simulink model "power_PSTdeltahex"  (Simulink 6.0)
settings: Solver=ode23tb  StartTime=0.0  StopTime=50  MaxStep=1/60  RelTol=1e-4  AbsTol=1e-3
undefined symbols (not defined in the file or in its folder): I21_init_imag, I21_init_real
libraries: powerlib x117, powerlib_extras x19, simulink_extras x1
(part 1 of 3)
settings Model: Creator=batserve  LastModifiedBy=batserve  ExtModeAutoUpdateStatusClock=off
settings DataIOCC: SignalLoggingName=sigsOut
settings DebuggingCC: CheckExecutionContextPreStartOutputMsg=on  CheckExecutionContextRuntimeOutputMsg=on  SolverPrmCheckMsg=none
settings HardwareCC: TargetUnknown=on

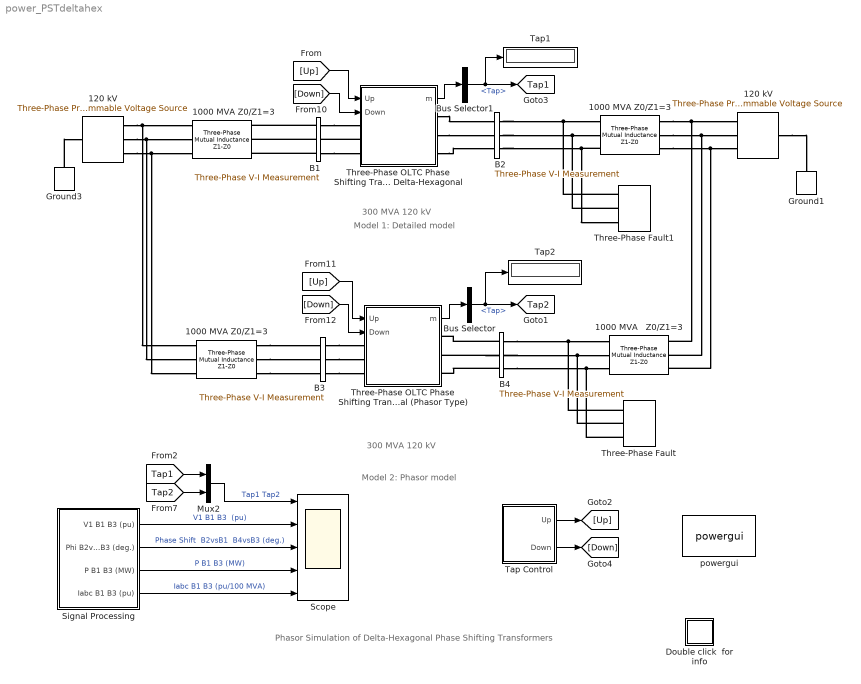
== system power_PSTdeltahex ==
  note: Phasor Simulation of Delta-Hexagonal Phase Shifting Transformers
  note: Model 1: Detailed model
  note: Model 2: Phasor model
  note: 300 MVA 120 kV
  note: 300 MVA 120 kV
  "1000 MVA Z0/Z1=3 " : powerlib/Elements/Three-Phase Mutual Inductance Z1-Z0  PhysicalDomain=powersysdomain  SubClassName=unknown  LeftPortType=p1  RightPortType=p1  LConnTagsString=a|b|c  RConnTagsString=A|B|C  PositiveSequence="[ 0.1  1/(2*pi*60)] *120e3^2/1000e6"  ZeroSequence="[ 0.3  3/(2*pi*60)] *120e3^2/1000e6"
  "1000 MVA Z0/Z1=3  " : powerlib/Elements/Three-Phase Mutual Inductance Z1-Z0  PhysicalDomain=powersysdomain  SubClassName=unknown  LeftPortType=p1  RightPortType=p1  LConnTagsString=a|b|c  RConnTagsString=A|B|C  PositiveSequence="[ 0.1  1/(2*pi*60)] *120e3^2/1000e6"  ZeroSequence="[ 0.3  3/(2*pi*60)] *120e3^2/1000e6"
  "1000 MVA Z0/Z1=3     " : powerlib/Elements/Three-Phase Mutual Inductance Z1-Z0  PhysicalDomain=powersysdomain  SubClassName=unknown  LeftPortType=p1  RightPortType=p1  LConnTagsString=a|b|c  RConnTagsString=A|B|C  PositiveSequence="[ 0.1  1/(2*pi*60)] *120e3^2/1000e6"  ZeroSequence="[ 0.3  3/(2*pi*60)] *120e3^2/1000e6"
  "1000 MVA   Z0/Z1=3       " : powerlib/Elements/Three-Phase Mutual Inductance Z1-Z0  PhysicalDomain=powersysdomain  SubClassName=unknown  LeftPortType=p1  RightPortType=p1  LConnTagsString=a|b|c  RConnTagsString=A|B|C  PositiveSequence="[ 0.1  1/(2*pi*60)] *120e3^2/1000e6"  ZeroSequence="[ 0.3  3/(2*pi*60)] *120e3^2/1000e6"
  120 kV : powerlib/Electrical Sources/Three-Phase Programmable Voltage Source  PositiveSequence=[120e3 0 60]  VariationEntity=None  VariationType=Table of time-amplitude pairs  VariationStep=0.2  VariationRate=10  VariationMagnitude=0.3  VariationFrequency=2  VariationTiming="[5  20]"  VariationPhaseA=off  Amplitudes="[ 1 0.95   1.1 ]"  TimeValues="[0  10 50]"  HarmonicGeneration=off  HarmonicA=[3 0.2 -25 0]  HarmonicB=[2 0.15 35 2]  Timing="[0.05  3]"
  "120 kV " : powerlib/Electrical Sources/Three-Phase Programmable Voltage Source  Orientation=left  PositiveSequence=[120e3 0 60]  VariationEntity=None  VariationType=Table of time-amplitude pairs  VariationStep=0.2  VariationRate=10  VariationMagnitude=0.3  VariationFrequency=2  VariationTiming="[5  20]"  VariationPhaseA=off  Amplitudes="[ 1 0.95   1.1 ]"  TimeValues="[0  10 50]"  HarmonicGeneration=off  HarmonicA=[3 0.2 -25 0]  HarmonicB=[2 0.15 35 2]  Timing="[0.05  3]"
  B1 : powerlib/Measurements/Three-Phase V-I Measurement  VoltageMeasurement=phase-to-ground  SetLabelV=on  LabelV=VabcB1  Vpu=on  Vbase=120e3  CurrentMeasurement=yes  SetLabelI=on  LabelI=IabcB1  Ipu=on  Pbase=100e6  OutputType=Complex  PhasorSimulation=on  PSBequivalent=0
  B2 : powerlib/Measurements/Three-Phase V-I Measurement  VoltageMeasurement=phase-to-ground  SetLabelV=on  LabelV=VabcB2  Vpu=on  Vbase=120e3  CurrentMeasurement=no  SetLabelI=on  LabelI=IB2  Ipu=off  Pbase=100e6  OutputType=Complex  PhasorSimulation=on  PSBequivalent=0
  B3 : powerlib/Measurements/Three-Phase V-I Measurement  VoltageMeasurement=phase-to-ground  SetLabelV=on  LabelV=VabcB3  Vpu=on  Vbase=120e3  CurrentMeasurement=yes  SetLabelI=on  LabelI=IabcB3  Ipu=on  Pbase=100e6  OutputType=Complex  PhasorSimulation=on  PSBequivalent=0
  B4 : powerlib/Measurements/Three-Phase V-I Measurement  VoltageMeasurement=phase-to-ground  SetLabelV=on  LabelV=VabcB4  Vpu=on  Vbase=120e3  CurrentMeasurement=no  SetLabelI=on  LabelI=IabcB4  Ipu=off  Pbase=100e6  OutputType=Complex  PhasorSimulation=on  PSBequivalent=0
  Bus Selector : BusSelector  DialogController=Simulink.DDGSource_Bus  OutputSignals=Tap
  Bus Selector1 : BusSelector  DialogController=Simulink.DDGSource_Bus  OutputSignals=Tap
  Double click  for info : Subsystem
      mask Display: disp('?')
  Ground1 : powerlib/Elements/Ground  Orientation=down  PhysicalDomain=powersysdomain  SubClassName=unknown  LeftPortType=p1  RightPortType=p1  LConnTagsString=a  RConnTagsString=__newr0
  Ground3 : powerlib/Elements/Ground  Orientation=down  PhysicalDomain=powersysdomain  SubClassName=unknown  LeftPortType=p1  RightPortType=p1  LConnTagsString=a  RConnTagsString=__newr0
  Mux2 : Mux  Inputs=2
  Scope : Scope  NumInputPorts=5
      settings: TimeRange=50  YMin=-5~0.94~-40~-400~0  YMax=5~1.02~40~400~3
  Signal Processing : Subsystem
      mask Display: disp('Signal\nProcessing')
  Tap Control : Subsystem
  Tap1 : Display
      settings: SampleTime=0.1
  Tap2 : Display
      settings: SampleTime=0.1
  Three-Phase Fault : powerlib/Elements/Three-Phase Fault  FaultA=off  FaultB=off  FaultC=off  FaultResistance=0.001  GroundFault=on  GroundResistance=0.001  External=off  SwitchStatus=[1 ]  SwitchTimes=[ 5 ]  InitialStates=[0 0 1]  SnubberResistance=1e6  SnubberCapacitance=inf  Measurements=None
  Three-Phase Fault1 : powerlib/Elements/Three-Phase Fault  FaultA=off  FaultB=off  FaultC=off  FaultResistance=0.001  GroundFault=on  GroundResistance=0.001  External=off  SwitchStatus=[1 ]  SwitchTimes=[ 5 ]  InitialStates=[0 0 1]  SnubberResistance=1e6  SnubberCapacitance=inf  Measurements=None
  Three-Phase OLTC Phase Shifting Transformer Delta-Hexagonal : Subsystem  mask(Phase Shifting Transformer; Delta-Hexagonal Connexion){NominalParameters=[120e3  300e6  60], RXpu=[0.15/30  0.15], RmXmpu=[500 500], SetSaturation=off, SaturationCurrentFlux=[0 0; 0.002 1.0; 0.006 1.12; 0.009 1.15; 0.015 1.17; 0.03 1.19; 0.05 1.20; 0.08 1.21; 1.0 1.302], InitialTap=0, TapSelectionTime=2.9, TransferTime=0.05, Rtransfer=1}
      mask prompts: NominalParameters "Nominal parameters [Vnom(Vrms Ph Ph) Pnom(VA)  Fnom(Hz)];"; RXpu "Resistance and leakage reactance at max. tap [R(pu)  X(pu)]"; RmXmpu "Magnetization branch [Rm(pu)  Xm(pu)]"; SetSaturation "Simulate saturation"; SaturationCurrentFlux "Saturation characteristic [i1 phi; i2 phi2; ....] (pu)"; InitialTap "Initial tap (-10 to +10)"; TapSelectionTime "Tap selection time (s) (typical 3-10 s)"; TransferTime "Tap transition time (s) (typical 40-60 ms)"; Rtransfer "Transfer resistances (ohms)"
      mask help:
      | This model implements a phase shifting transformer (PST) using the delta-hexagonal connexion. Each phase consists of two coupled windings: one fixed winding and one tapped winding (10 taps per half winding or 21 taps total). Two OLTCs are used to vary phase shift from -60 degrees to + 60 degrees by moving the transformer input connections (ABC) and output connections (abc) symmetrically  with respect to center of the tapped winding. The OLTCs move taps one step upward or downward when the signals connected to the "Up" and "Down" inputs change from 0 to 1.
      |
      | For equally spaced taps, phase shift of output voltages (abc) with respect to input voltages (ABC) varies as follows:
      |     Psi= 2*atan(-tap/10/sqrt(3))
      | where:
      |    tap= position of the 2 OLTCs (-10<= tap<= 10)
      |
      | Tap = [0    1      2        3        4         5       6      7       8       9        10  ]
      | Phi  = [0   -6.6  -13.2  -19.7  -26.0  -32.2 -38.2 -44.0 -49.6.-54.9  -60.0]
      mask init:
      | NumberOfTaps=10;
      | if abs(InitialTap)>NumberOfTaps,
      |    h=errordlg(sprintf('The initial tap number must be an integer comprised between % d and %d',-NumberOfTaps,NumberOfTaps),'Parameter error');
      |    uiwait(h);
      | end
      | 
      | % Saturation
      | set_param([gcb,'/TransfoA'],'SetSaturation',SetSaturation);
      | set_param([gcb,'/TransfoB'],'SetSaturation',SetSaturation);
      | set_param([gcb,'/TransfoC'],'SetSaturation',SetSaturation);
      mask CallbackString:
      | |||tempMaskVis=get_param(gcb,'MaskVisibilities');
      | if strcmp(get_param(gcb,'SetSaturation'),'on')
      | 	tempMaskVis{5}='on';
      | 	set_param(gcb,'MaskVisibilities',tempMaskVis);
      | else
      | 	tempMaskVis{5}='off';
      | 	set_param(gcb,'MaskVisibilities',tempMaskVis);
      | end|||||
  Three-Phase OLTC Phase Shifting Transformer Delta-Hexagonal (Phasor Type) : Subsystem  mask(Phase Shifting Transformer; Delta-Hexagonal Connexion (phasor)){NominalParameters=[120e3  300e6  60], RXpu=[0.15/30  0.15], RXm=[500 500], NumberOfTaps=10, InitialTap=0, TapSelectionTime=2.9, Iout_init=[ 0  0]}
      mask prompts: NominalParameters "Nominal parameters [Vnom(Vrms Ph Ph) Pnom(VA)  Fnom(Hz)];"; RXpu "Resistance and leakage reactance at max. tap [R(pu)  X(pu)]"; RXm "Magnetization branch [Rm(pu)  Xm(pu)]"; NumberOfTaps "Number of taps per half tapped winding"; InitialTap "Initial tap"; TapSelectionTime "Tap selection time (s) (typical 3-10 s)"; Iout_init "Initial pos. seq. of output currents [Mag(pu)  Phase(deg)]"
      mask help:
      | This model implements a phasor model of a phase shifting transformer (PST) using the delta-hexagonal connexion. Each phase consists of two coupled windings: one fixed winding and one tapped winding. Two OLTCs are used to vary phase shift from -60 degrees to + 60 degrees
      | by moving the transformer input connections (ABC) and output connections (abc) symmetrically with respect to center of the tapped winding. The OLTCs move taps one step upward or downward when the signals connected to the "Up" and "Down" inputs change from 0 to 1.
      |
      | Phase shift Psi of output voltages (abc) with respect to input voltages (ABC) varies as follows:
      |     Psi= 2*atan(-k/sqrt(3))
      | where:
      |    k= tap position of the 2 OLTCs with respect to center of tapped winding
      |         k= tap/NumberOfTaps  ( -1<= k<= 1)
      |    k=0 indicates taps at winding mid point (Psi=0)
      |    k= 1 --> Psi=-60 deg;  k=-1--> Psi = -60 deg.
      mask init:
      | if abs(InitialTap)>NumberOfTaps
      |    h=errordlg(sprintf('The initial tap number must be an integer comprised between % d and %d',-NumberOfTaps,NumberOfTaps),'Parameter error');
      |    uiwait(h);
      | end
      | Vnom=NominalParameters(1);
      | Pnom=NominalParameters(2);
      | Fnom=NominalParameters(3);
      | w=2*pi*Fnom;
      | Ibase=Pnom/Vnom/sqrt(3)*sqrt(2);
      | 
      | TapMinMax=[-NumberOfTaps NumberOfTaps];
      | 
      | j=sqrt(-1);
      | a=exp(j*2*pi/3);
      | Z1pu=RXpu(1)+j*RXpu(2);     % Impedance at max tap position
      | Zmpu=(RXm(1)*j*RXm(2))/(RXm(1)+j*RXm(2)); % Magnetization Impedance at max tap position
      | 
      | I2_init_mag=Iout_init(1); % Mag pos. seq. (pu)
      | I2_init_pha=Iout_init(2); % Phase pos. seq. (deg)
      | I2A_init_mag=I2_init_mag*Ibase;
      | I2B_init_mag=I2_init_mag*Ibase;
      | I2C_init_mag=I2_init_mag*Ibase;
      | I2A_init_pha=I2_init_pha;
      | I2B_init_pha=I2_init_pha-120;
      | I2C_init_pha=I2_init_pha+120;
      | 
      | psi=2*atan(-InitialTap/NumberOfTaps/sqrt(3))*180/pi; % degrees
      | 
      | I1A_init_mag=I2A_init_mag;
      | I1B_init_mag=I2B_init_mag;
      | I1C_init_mag=I2C_init_mag;
      | I1A_init_pha=I2A_init_pha-psi;
      | I1B_init_pha=I2B_init_pha-psi;
      | I1C_init_pha=I2C_init_pha-psi;
      | 
      | %Initialisation of pos. seq. transfer functions for breaking alg. loop
      | [I21_init_real, I21_init_imag]=pol2cart(I2_init_pha*pi/180,I2_init_mag);
  powergui : powerlib/powergui  Priority=2  Frange=[0:2:500]  Ylog=off  Xlog=on  save=off  variable=ZData  ZoomFFT=on  StartTime=0.0  cycles=1  DisplayStyle=1  fundamental=60  FreqAxis=off  MaxFrequency=1000  frequencyindice=1  frequencyindicesteady=1  RmsSteady=2  display=off  Ts=0  methode=on  frequency=60  echomessages=off
  tag scope: Tap1=global, Tap2=global
  wires:
  [Tap1] -> Mux2/1
  [Tap2] -> Mux2/2
  Mux2/1 -> Scope/1  "Tap1 Tap2"
  Tap Control/1(Up) -> [Up]
  Tap Control/2(Down) -> [Down]
  Signal Processing/4(Iabc B1 B3 (pu)) -> Scope/5  "Iabc B1 B3 (pu/100 MVA)"
  Signal Processing/1(V1 B1 B3 (pu)) -> Scope/2  "V1 B1 B3  (pu)"
  Signal Processing/2(Phi B2vsB1  B4vsB3 (deg.)) -> Scope/3  "Phase Shift  B2vsB1  B4vsB3 (deg.)"
  Signal Processing/3(P B1 B3 (MW)) -> Scope/4  "P B1 B3 (MW)"
  Three-Phase OLTC Phase Shifting Transformer Delta-Hexagonal (Phasor Type)/1(m) -> Bus Selector/1
  Bus Selector/1 -> [Tap2], Tap2/1  "<Tap>"
  Three-Phase OLTC Phase Shifting Transformer Delta-Hexagonal/1(m) -> Bus Selector1/1
  Bus Selector1/1 -> [Tap1], Tap1/1  "<Tap>"
  [Down] -> Three-Phase OLTC Phase Shifting Transformer Delta-Hexagonal/2(Down)
  [Down] -> Three-Phase OLTC Phase Shifting Transformer Delta-Hexagonal (Phasor Type)/2(Down)
  [Up] -> Three-Phase OLTC Phase Shifting Transformer Delta-Hexagonal (Phasor Type)/1(Up)
  [Up] -> Three-Phase OLTC Phase Shifting Transformer Delta-Hexagonal/1(Up)
  connections:
  Three-Phase OLTC Phase Shifting Transformer Delta-Hexagonal/LConn2 -- B1/RConn2
  Ground3/LConn1 -- 120 kV/LConn1
  B1/RConn1 -- Three-Phase OLTC Phase Shifting Transformer Delta-Hexagonal/LConn1
  B1/RConn3 -- Three-Phase OLTC Phase Shifting Transformer Delta-Hexagonal/LConn3
  B3/RConn1 -- Three-Phase OLTC Phase Shifting Transformer Delta-Hexagonal (Phasor Type)/LConn1
  B3/RConn2 -- Three-Phase OLTC Phase Shifting Transformer Delta-Hexagonal (Phasor Type)/LConn2
  B3/RConn3 -- Three-Phase OLTC Phase Shifting Transformer Delta-Hexagonal (Phasor Type)/LConn3
  B1/LConn1 -- "1000 MVA Z0/Z1=3 "/RConn1
  B1/LConn2 -- "1000 MVA Z0/Z1=3 "/RConn2
  B1/LConn3 -- "1000 MVA Z0/Z1=3 "/RConn3
  "1000 MVA Z0/Z1=3  "/RConn1 -- B3/LConn1
  "1000 MVA Z0/Z1=3  "/RConn2 -- B3/LConn2
  "1000 MVA Z0/Z1=3  "/RConn3 -- B3/LConn3
  "1000 MVA   Z0/Z1=3       "/RConn1 -- "120 kV "/RConn1 -- "1000 MVA Z0/Z1=3     "/RConn1
  "120 kV "/LConn1 -- Ground1/LConn1
  "1000 MVA   Z0/Z1=3       "/RConn2 -- "120 kV "/RConn2 -- "1000 MVA Z0/Z1=3     "/RConn2
  "1000 MVA   Z0/Z1=3       "/RConn3 -- "120 kV "/RConn3 -- "1000 MVA Z0/Z1=3     "/RConn3
  Three-Phase OLTC Phase Shifting Transformer Delta-Hexagonal/RConn2 -- B2/LConn2
  Three-Phase OLTC Phase Shifting Transformer Delta-Hexagonal/RConn1 -- B2/LConn1
  Three-Phase OLTC Phase Shifting Transformer Delta-Hexagonal/RConn3 -- B2/LConn3
  B4/LConn1 -- Three-Phase OLTC Phase Shifting Transformer Delta-Hexagonal (Phasor Type)/RConn1
  B4/LConn2 -- Three-Phase OLTC Phase Shifting Transformer Delta-Hexagonal (Phasor Type)/RConn2
  B4/LConn3 -- Three-Phase OLTC Phase Shifting Transformer Delta-Hexagonal (Phasor Type)/RConn3
  120 kV/RConn1 -- "1000 MVA Z0/Z1=3 "/LConn1 -- "1000 MVA Z0/Z1=3  "/LConn1
  120 kV/RConn2 -- "1000 MVA Z0/Z1=3 "/LConn2 -- "1000 MVA Z0/Z1=3  "/LConn2
  120 kV/RConn3 -- "1000 MVA Z0/Z1=3 "/LConn3 -- "1000 MVA Z0/Z1=3  "/LConn3
  Three-Phase Fault/LConn3 -- "1000 MVA   Z0/Z1=3       "/LConn3 -- B4/RConn3
  Three-Phase Fault/LConn2 -- "1000 MVA   Z0/Z1=3       "/LConn2 -- B4/RConn2
  Three-Phase Fault/LConn1 -- "1000 MVA   Z0/Z1=3       "/LConn1 -- B4/RConn1
  B2/RConn3 -- "1000 MVA Z0/Z1=3     "/LConn3 -- Three-Phase Fault1/LConn3
  B2/RConn1 -- Three-Phase Fault1/LConn1 -- "1000 MVA Z0/Z1=3     "/LConn1
  B2/RConn2 -- Three-Phase Fault1/LConn2 -- "1000 MVA Z0/Z1=3     "/LConn2

== system power_PSTdeltahex/Double click  for info ==
  note: This demonstration illustrates operation of two models of Phase Shifting Transformer (PST) using On Load Tap Changers (OLTC)
  note: Circuit Description
  note: Two 120 kV 1000 MVA networks are interconnected through a phase shifting transformer (PST) . The phase shift can be varied on load  by means of On Load Tap Changers (OLTC).
      | The same circuit is duplicated in order to compare the performance of  two different models of PST:
      |
      |     - Model 1 is a detailed model where all OLTC switches and transformer characteristics are represented. This model can be used with either continuous or discrete
      |        solvers to get detailed waveshapes or with the phasor simulation method to observe variations of  phasor voltages and currents.
      |     - Model 2 is a simplified phasor model where the transformer and the OLTCs are simulated by current sources. This model can be used only with the phasor solution method
      |        The phasor model is much faster to execute and it should be the preferred model for transient stability studies.
      |
      | Both models implement a three-phase phase PST rated 120 kV, 300 MVA, and using the delta-hexagonal connection.
      | The PSTs are used to control the power transferred between the two 120 kV networks.
      |
      | Each phase consists of two coupled windings (one winding without taps, and one tapped winding). Two OLTCs are used to vary phase shift  from -60 degrees to + 60 degrees
      | by moving the transformer input connections (ABC) and  output connections (abc) symmetrically  with respect to center of the tapped winding. Each OLTC consists of ten (10)
      | switches allowing selection of  tap position -10 to +10. Taps +10 and -10 provide respectively -60 degrees and + 60 degrees phase shift of abc voltages with respect to ABC,
      | while tap 0 provides zero phase shift. With 10 taps per half winding, each tap provides approximately 6 degrees phase shift. The phase shift variation as function of tap position
      | is given in the block menu. When pulses are sent at the "Up" or  "Down" inputs, the taps move either in the positive or negative direction.
      |
      | Open the two PST block menus and look at  their parameters. The detailed model is buit with a fixed number of taps (10) whereas the phasor model allows specifying any number
      | of taps. Simulation of saturation is permitted with the detailed model only, providing that a phasor solution method is not used (specify "Continuous" or "Discretize electrical model"
      | in the powergui block).
      |
      | You can also use 'Edit/Look under mask' to see how the transformer models are built. The detailed model is built from three Multi-Winding Transformer blocks and
      | three OLTC subsystems which contain switches performing  tap selection and reversal of the regulation winding. The tap transition is performed by temporarily
      | short-circuiting two adjacent transformer taps through resistors (1 ohm resistances and 50 ms transition time as specified in the block menu of the detailed model).
      | The phasor model is built with current sources emulating the transformer impedance which depends on winding resistances, leakage reactances and tap position.
  note: G. Sybille (Hydro-Quebec)
  note: In order to observe impact of phase shift on power transfer, the phase shift is increased from zero to 32.2 degrees lagging (tap +5), then phase shift is reduced
      | to zero and increased again up to 32.2 degrees leading. This is performed by sending 5 pulses to the "Up" input, and then, 10 pulses to the "Down" input ".
      | As the tap selection is a relatively slow mechanical process (3 sec per tap as specified in the "Tap selection time" parameter of the block menus), the simulation Stop time
      | is set to 50 s.
      |
      | Start simulation and observe PST operation on the Scope. Results obtained with the two models are superimposed on five traces.
      | Trace 1 shows the tap position. Trace 2 shows a superposition of positive-sequence voltages measured at bus B1 (yellow) and bus B3 (magenta) .
      | Traces 3 shows the phase shifts of positive-sequence voltages measured at output terminals (abc) with respect to input terminals (ABC).
      | Trace 4 compares the active power measured at bus B1(yellow) and bus B3 (magenta). Trace 5 ...
      |
      | When simulation starts the OLTCs are at position 0 (zero phase shift).  As the two networks are symmetrical with both internal angles set at 0 degree,  there is no current flowing.
      | Then, phase shift is increased and bus B2 (or  B4) is lagging bus B1(or B3).  As B2 is lagging the internal voltage of the source located on right side, power flows from
      | right to left. Power measured from left to right is therefore negative for positive tap positions.
      | The maximum power is obtained at tap +5, or -5 when the phase shift is respectively -32.2 degrees and +32.2 degrees.
      | The active power can be computed from P= V1.V2*sin(psi)/ (X1 +X2 + Xpst) , where: V1=V2=internal voltages= 1.0 pu ;  X1= X2 = network reactances =  1pu /1000 MVA
      | Xpst= PST leakage reactance at tap 5. The PST leakage reactance varies vith tap position (from zero at tap zero to 0.15 pu at maximum tap (10)).
      | The positive-sequence impedance of the phasor model is available as a signal at its measurement output "m". The reactance obtained at tap 5 is  Xpst=0.1067 pu/ 300 MVA.
      | The total reactance expressed in pu/100 MVA is X= 0.1 +0.1 + 0.1067/3 =0.2356 pu/100 MVA.
      | The expected active power at tap 5 is P= 1*sin(32.2deg)/0.2356 = 2.26 pu/100 MVA or 226 MW, which corresponds well with the measured value on trace 4 (224 MW)
      | Because of the voltage developed across the PST leakage reactance, the phase shift measured between PST input and output voltages (trace 3) is lower than the expected value.
      | For example, 27.2 degrees is obtained at tap 5, instead of the 32.2 degrees theoretical value computed at no load. The phase shift variation depends on load current.
  note: Demonstration
  note: Simulation with phasor model only
  note: In order to appreciate the gain in simulation speed provided by the phasor model, delete the detailed PST model and replace it with a duplicate of the phasor model.
      | Reconnect control signals to the "Up" and  "Down" inputs. Restart simulation. The model runs approximately 5 times faster, mainly because the OLTC switches of the
      | detailed model are not simulated.
  note: Open loop control of power transfer
  note: Initializating the phasor model
  note: For the phasor model to start initialized at t=0, the current sources used in the model must be inialized with current values corresponding to steady state.
      | Suppose that you want to start with the initial tap position 5. First, in the two block menus, "set Initial tap" parameter to 5. Then disconnect the signals connected to the
      | "Up" and   "Down" inputs of the two models, so that the taps stay at position 5.  If you start simulation you will notice a transient in the phasor model signals at  t=0 because
      | the model is not initialized. Use the "Steady-State Voltages and Currents" option of the powergui to obtain the initial current flowing in the detailed model at bus B4.
      | The phase  A output current identified "B2/Ia" is 1129.4 A rms, 169 degrees. This current converted to per unit based on PST rating is 1129/1443 = 0.7824 pu/ 300MVA.
      | Specify [ 0.7824 169]  in the "Initial pos. seq. output current" parameter. If you now restart simulation, you should observe no transient at t=0.
  note: Operation under unbalanced conditions
  note: The phasor model is valid for unbalanced conditions. If you check "Phase A Fault" in the the two fault breakers, a single-phase fault will be applied at t=5s.
      | The currents measured at buses B1and B3 should be identical. (Ia=3.48 pu, Ib=2.25 pu  Ic=2.10 pu at tap position +5).

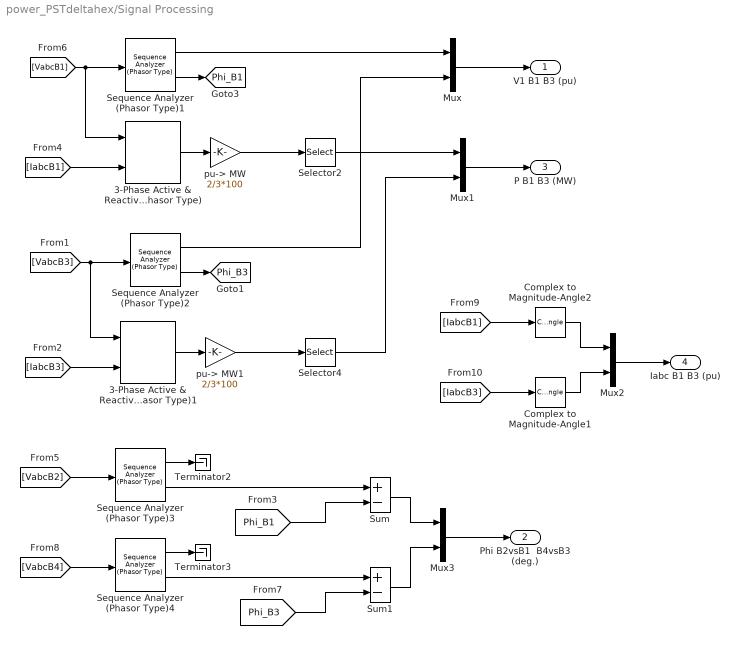
== system power_PSTdeltahex/Signal Processing ==
  3-Phase Active & Reactive Power (Phasor Type) : powerlib_extras/Phasor Library/3-Phase Active & Reactive Power (Phasor Type)
  3-Phase Active & Reactive Power (Phasor Type)1 : powerlib_extras/Phasor Library/3-Phase Active & Reactive Power (Phasor Type)
  Complex to Magnitude-Angle1 : ComplexToMagnitudeAngle  Output=Magnitude
  Complex to Magnitude-Angle2 : ComplexToMagnitudeAngle  Output=Magnitude
  Mux{,1..3} (4 alike) : Mux  Inputs=2
  Selector2 : Selector  InputPortWidth=2
  Selector4 : Selector  InputPortWidth=2
  Sequence Analyzer (Phasor Type){1..4} (4 alike) : powerlib_extras/Phasor Library/Sequence Analyzer (Phasor Type)  seq=Positive
  Sum : Sum  Inputs=+-  SaturateOnIntegerOverflow=on
  Sum1 : Sum  Inputs=+-  SaturateOnIntegerOverflow=on
  Terminator2 : Terminator
  Terminator3 : Terminator
  pu-> MW : Gain  Gain=2/3*100  SaturateOnIntegerOverflow=on
  pu-> MW1 : Gain  Gain=2/3*100  SaturateOnIntegerOverflow=on
  V1 B1 B3 (pu) : Outport
  Phi B2vsB1  B4vsB3 (deg.) : Outport  Port=2
  P B1 B3 (MW) : Outport  Port=3
  Iabc B1 B3 (pu) : Outport  Port=4
  tag scope: Phi_B1=global, Phi_B3=global
  wires:
  [VabcB1] -> Sequence Analyzer (Phasor Type)1/1, 3-Phase Active & Reactive Power (Phasor Type)/1
  Sequence Analyzer (Phasor Type)1/2 -> [Phi_B1]
  3-Phase Active & Reactive Power (Phasor Type)/1 -> pu-> MW/1
  3-Phase Active & Reactive Power (Phasor Type)1/1 -> pu-> MW1/1
  pu-> MW/1 -> Selector2/1
  pu-> MW1/1 -> Selector4/1
  [VabcB3] -> Sequence Analyzer (Phasor Type)2/1, 3-Phase Active & Reactive Power (Phasor Type)1/1
  Sequence Analyzer (Phasor Type)2/1 -> Mux/2
  Sequence Analyzer (Phasor Type)2/2 -> [Phi_B3]
  [IabcB1] -> 3-Phase Active & Reactive Power (Phasor Type)/2
  [IabcB3] -> 3-Phase Active & Reactive Power (Phasor Type)1/2
  Sequence Analyzer (Phasor Type)1/1 -> Mux/1
  Mux/1 -> V1 B1 B3 (pu)/1
  Mux1/1 -> P B1 B3 (MW)/1
  Selector2/1 -> Mux1/1
  Selector4/1 -> Mux1/2
  Sequence Analyzer (Phasor Type)3/2 -> Sum/1
  [Phi_B1] -> Sum/2
  Sequence Analyzer (Phasor Type)3/1 -> Terminator2/1
  [VabcB2] -> Sequence Analyzer (Phasor Type)3/1
  Sequence Analyzer (Phasor Type)4/2 -> Sum1/1
  [Phi_B3] -> Sum1/2
  Sequence Analyzer (Phasor Type)4/1 -> Terminator3/1
  [VabcB4] -> Sequence Analyzer (Phasor Type)4/1
  Sum/1 -> Mux3/1
  Sum1/1 -> Mux3/2
  Mux3/1 -> Phi B2vsB1  B4vsB3 (deg.)/1
  [IabcB1] -> Complex to Magnitude-Angle2/1
  Complex to Magnitude-Angle2/1 -> Mux2/1
  Mux2/1 -> Iabc B1 B3 (pu)/1
  [IabcB3] -> Complex to Magnitude-Angle1/1
  Complex to Magnitude-Angle1/1 -> Mux2/2

== system power_PSTdeltahex/Tap Control ==
  Product : Product  SaturateOnIntegerOverflow=on
  Product1 : Product  SaturateOnIntegerOverflow=on
  Pulse Generator : DiscretePulseGenerator  PulseType=Time based  Period=3  PulseWidth=5
  Pulse Generator1 : DiscretePulseGenerator  PulseType=Time based  Period=3  PulseWidth=5
  Timer1 : powerlib_extras/Control  Blocks/Timer  t="[ 0  16   ]"  e="[1   0   ]"
  Timer2 : powerlib_extras/Control  Blocks/Timer  t="[ 0  17  47 ]"  e="[0  1   0  ]"
  Up : Outport
  Down : Outport  Port=2
  wires:
  Pulse Generator/1 -> Product/1
  Timer1/1 -> Product/2
  Pulse Generator1/1 -> Product1/1
  Timer2/1 -> Product1/2
  Product1/1 -> Down/1
  Product/1 -> Up/1

== system power_PSTdeltahex/Three-Phase OLTC Phase Shifting Transformer Delta-Hexagonal ==
  Up : Inport  Port=1  LatchInput=off
  Down : Inport  Port=2  LatchInput=off
  Goto Tag Visibility : GotoTagVisibility  GotoTag=SwSelect
  Goto Tag Visibility1 : GotoTagVisibility  GotoTag=SwTransfer
  Goto Tag Visibility2 : GotoTagVisibility  GotoTag=SwInversion
  Mux : Mux  Inputs=2
  OLTC Control : Subsystem  mask{NumberOfTaps=NumberOfTaps, TapSelectorTime=TapSelectionTime, TransferSwitchTime=TransferTime, InitialTap=InitialTap}
      mask prompts: NumberOfTaps "Number of taps:"; TapSelectorTime "Operating time of the tap selector (typical 3-10 s):"; TransferSwitchTime "Operating time of the transfer switch (typical 40-60 ms):"; InitialTap "Initial tap:"
      mask init:
      | TapVector=0:2*NumberOfTaps;
      | InitialStates1=zeros(1,2*NumberOfTaps+1);
      | InitialStates1(NumberOfTaps+abs(InitialTap)+1)=1;
      | InitialStates2=zeros(1,2*NumberOfTaps+1);
      | InitialStates2(NumberOfTaps-abs(InitialTap)+1)=1;
  Subsystem1 : Subsystem
      mask Display: disp('Double click\nto see\nTransforner\nConnections')
  TransfoA : Subsystem  mask{NominalParameters=NominalParameters, RXpu=RXpu, RmXmpu=RmXmpu, SetSaturation=off, SaturationCurrentFlux=SaturationCurrentFlux, NumberOfTaps=NumberOfTaps, InitialTap=InitialTap, R=Rtransfer}
      mask prompts: NominalParameters "Nominal parameters [Vnom(Vrms Ph Ph) Pnom(VA)  Fnom(Hz)];"; RXpu "Resistance and leakage reactance at max. tap [R(pu)  X(pu)]"; RmXmpu "Magnetization branch [Rm(pu)  Xm(pu)]"; SetSaturation "Simulate saturation"; SaturationCurrentFlux "Saturation characteristic [i1 phi; i2 phi2; ....] (pu)"; NumberOfTaps "Number of taps"; InitialTap "Initial tap (-10 to +10)"; R "Transfer resistances (ohms)"
      mask init:
      | VnomLL=NominalParameters(1); % Tension LL nominale
      | Pnom3ph=NominalParameters(2);
      | Fnom=NominalParameters(3);
      | N=NumberOfTaps*2;
      | Ron=1e-4; % Resistance des interrupteurs
      | Rsnub=1e6;% Resistance des snubbers aux bornes des interrupteurs
      | 
      | % Tension nominale de chaque enroulement
      | % = Tension max. par enroulement obtenu a la prise 0
      | % =VLN_nom*2/sqrt(3)  --> Vnominal enroulements=Vnom*2/3 
      | Vnom_Windings=[VnomLL*2/3, VnomLL*2/3];
      | % RXpu= R et X des 2 enroulements en pu sur Pnom3ph et VnomLL
      | % RXpunom= R et X de chaque enroulement 
      | % en pu sur tension nominale des enroulements (VnomLL*2/3)  et Pnom3ph/3
      | RXpunom=RXpu/2*9/4; 
      | Rpu_Windings=[RXpunom(1), RXpunom(1)];
      | Xpu_Windings=[RXpunom(2), RXpunom(2)];
      | 
      | % RmXmpu= Rm et Xm en pu sur tension nominale des enroulements (VnomLL*2/3)et Pnom3ph/3  
      | Rmag=RmXmpu(1);
      | Lmag=RmXmpu(2);
      | 
      | % Saturation
      | set_param([gcb,'/Transformer'],'SetSaturation',SetSaturation)
      | 
      | InitialStates1=zeros(1,N+1);
      | InitialStates1(NumberOfTaps+abs(InitialTap)+1)=1;
      | InitialStates2=zeros(1,N+1);
      | InitialStates2(NumberOfTaps-abs(InitialTap)+1)=1;
      | InitialStates=InitialStates1|InitialStates2;
  TransfoB : Subsystem  mask{NominalParameters=NominalParameters, RXpu=RXpu, RmXmpu=RmXmpu, SetSaturation=off, SaturationCurrentFlux=SaturationCurrentFlux, NumberOfTaps=NumberOfTaps, InitialTap=InitialTap, R=Rtransfer}
      mask prompts: NominalParameters "Nominal parameters [Vnom(Vrms Ph Ph) Pnom(VA)  Fnom(Hz)];"; RXpu "Resistance and leakage reactance at max. tap [R(pu)  X(pu)]"; RmXmpu "Magnetization branch [Rm(pu)  Xm(pu)]"; SetSaturation "Simulate saturation"; SaturationCurrentFlux "Saturation characteristic [i1 phi; i2 phi2; ....] (pu)"; NumberOfTaps "Number of taps"; InitialTap "Initial tap (-10 to +10)"; R "Transfer resistances (ohms)"
      mask init: same as power_PSTdeltahex/Three-Phase OLTC Phase Shifting Transformer Delta-Hexagonal/TransfoA
  TransfoC : Subsystem  mask{NominalParameters=NominalParameters, RXpu=RXpu, RmXmpu=RmXmpu, SetSaturation=off, SaturationCurrentFlux=SaturationCurrentFlux, NumberOfTaps=NumberOfTaps, InitialTap=InitialTap, R=Rtransfer}
      mask prompts: NominalParameters "Nominal parameters [Vnom(Vrms Ph Ph) Pnom(VA)  Fnom(Hz)];"; RXpu "Resistance and leakage reactance at max. tap [R(pu)  X(pu)]"; RmXmpu "Magnetization branch [Rm(pu)  Xm(pu)]"; SetSaturation "Simulate saturation"; SaturationCurrentFlux "Saturation characteristic [i1 phi; i2 phi2; ....] (pu)"; NumberOfTaps "Number of taps"; InitialTap "Initial tap (-10 to +10)"; R "Transfer resistances (ohms)"
      mask init: same as power_PSTdeltahex/Three-Phase OLTC Phase Shifting Transformer Delta-Hexagonal/TransfoA
  A : PMIOPort  Tag=PMCPort  Port=1  Side=Left
  B : PMIOPort  Tag=PMCPort  Port=2  Side=Left
  C : PMIOPort  Tag=PMCPort  Port=3  Side=Left
  a : PMIOPort  Tag=PMCPort  Orientation=left  Port=4  Side=Right
  b : PMIOPort  Tag=PMCPort  Orientation=left  Port=5  Side=Right
  c : PMIOPort  Tag=PMCPort  Orientation=left  Port=6  Side=Right
  m : Outport
  tag scope: SwInversion=scoped, SwSelect=scoped, SwTransfer=scoped
  wires:
  OLTC Control/4(SwTr) -> [SwTransfer]
  OLTC Control/3(SwSelect) -> [SwSelect]
  OLTC Control/5(SwInv) -> [SwInversion]
  Up/1 -> OLTC Control/1(Up)
  Down/1 -> OLTC Control/2(Down)
  Mux/1 -> m/1
  OLTC Control/1(Tap) -> Mux/1  "Tap"
  OLTC Control/2(Ready) -> Mux/2  "Ready"
  connections:
  TransfoA/RConn1 -- TransfoC/RConn3
  TransfoC/LConn3 -- TransfoB/LConn1
  TransfoA/LConn3 -- TransfoC/LConn1
  C/RConn1 -- TransfoC/LConn2
  TransfoB/RConn2 -- b/RConn1
  TransfoC/RConn2 -- c/RConn1
  TransfoA/LConn1 -- TransfoB/LConn3
  TransfoA/RConn2 -- a/RConn1
  TransfoB/RConn1 -- TransfoA/RConn3
  A/RConn1 -- TransfoA/LConn2
  B/RConn1 -- TransfoB/LConn2
  TransfoB/RConn3 -- TransfoC/RConn1

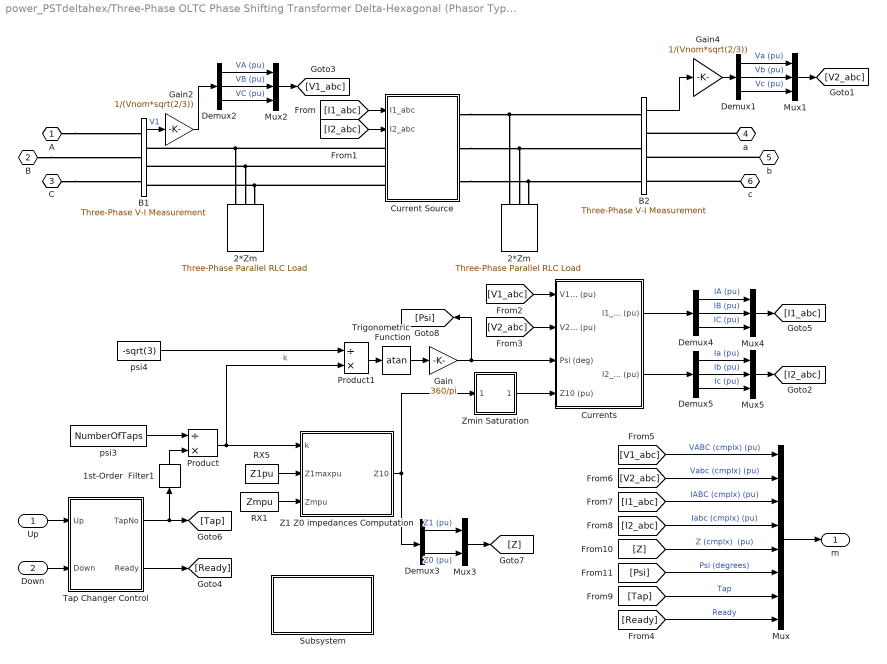
== system power_PSTdeltahex/Three-Phase OLTC Phase Shifting Transformer Delta-Hexagonal (Phasor Type) ==
  Up : Inport  Port=1  LatchInput=off
  Down : Inport  Port=2  LatchInput=off
  " Currents" : Subsystem
  1st-Order  Filter1 : powerlib_extras/Control  Blocks/1st-Order  Filter  Orientation=up  FilterType=Lowpass  Tc=1/Fnom  Initialize=on  Vac_Init="[0 0  Fnom]"  Vdc_Init=InitialTap  PlotResponse=off  param1=[1 500 1]
  2*Zm : powerlib/Elements/Three-Phase Parallel RLC Load  Orientation=down  PhysicalDomain=powersysdomain  SubClassName=unknown  LeftPortType=p1  RightPortType=p1  LConnTagsString=A|B|C  Configuration=Y (grounded)  NominalVoltage=Vnom  NominalFrequency=60  ActivePower=Pnom/RXm(1)/2  InductivePower=Pnom/RXm(2)/2  CapacitivePower=0  Measurements=None
  "2*Zm " : powerlib/Elements/Three-Phase Parallel RLC Load  Orientation=down  PhysicalDomain=powersysdomain  SubClassName=unknown  LeftPortType=p1  RightPortType=p1  LConnTagsString=A|B|C  Configuration=Y (grounded)  NominalVoltage=Vnom  NominalFrequency=60  ActivePower=Pnom/RXm(1)/2  InductivePower=Pnom/RXm(2)/2  CapacitivePower=0  Measurements=None
  B1 : powerlib/Measurements/Three-Phase V-I Measurement  VoltageMeasurement=phase-to-ground  SetLabelV=off  LabelV=Vabc_B21  Vpu=off  Vbase=25e3  CurrentMeasurement=no  SetLabelI=off  LabelI=Iabc_B21  Ipu=off  Pbase=10e6  OutputType=Complex  PhasorSimulation=on  PSBequivalent=0
  B2 : powerlib/Measurements/Three-Phase V-I Measurement  VoltageMeasurement=phase-to-ground  SetLabelV=off  LabelV=Vabc_B21  Vpu=off  Vbase=25e3  CurrentMeasurement=no  SetLabelI=off  LabelI=Iabc_B21  Ipu=off  Pbase=10e6  OutputType=Complex  PhasorSimulation=on  PSBequivalent=0
  Current Source : Subsystem
  Demux{1..2,4..5} (4 alike) : Demux  Outputs=3
  Demux3 : Demux  Outputs=2
  Gain : Gain  Gain=360/pi  SaturateOnIntegerOverflow=on
  Gain2 : Gain  Gain=1/(Vnom*sqrt(2/3))  SaturateOnIntegerOverflow=on
  Gain4 : Gain  Gain=1/(Vnom*sqrt(2/3))  SaturateOnIntegerOverflow=on
  Mux : Mux  Inputs=8
  Mux{1..2,4..5} (4 alike) : Mux  Inputs=3
  Mux3 : Mux  Inputs=2
  Product : Product  Inputs=/*  SaturateOnIntegerOverflow=on
  Product1 : Product  Inputs=/*  SaturateOnIntegerOverflow=on
  RX1 : Constant  Value=Zmpu
  RX5 : Constant  Value=Z1pu
  Subsystem : Subsystem
      mask Display: disp('Double click\nfor\ninfo')
  Tap Changer Control : Subsystem  mask(Tap Changer Control){MinMaxTap=TapMinMax, InitialPosition=InitialTap, MecDelay=TapSelectionTime}
      mask prompts: MinMaxTap "Minimum and maximum tap number [ Min  Max ] :"; InitialPosition "Initial tap position"; MecDelay "Mechanical delay time"
      mask init:
      | if MecDelay<=0,
      | 	MecDelay=1/60;
      | end
  Trigonometric Function : Trigonometry  Operator=atan
  "Z1 Z0 impedances Computation " : Subsystem
  Zmin Saturation : Subsystem
  psi3 : Constant  Value=NumberOfTaps
  psi4 : Constant  Value=-sqrt(3)
  A : PMIOPort  Tag=PMCPort  Port=1  Side=Left
  B : PMIOPort  Tag=PMCPort  Port=2  Side=Left
  C : PMIOPort  Tag=PMCPort  Port=3  Side=Left
  a : PMIOPort  Tag=PMCPort  Orientation=left  Port=4  Side=Right
  b : PMIOPort  Tag=PMCPort  Orientation=left  Port=5  Side=Right
  c : PMIOPort  Tag=PMCPort  Orientation=left  Port=6  Side=Right
  m : Outport
  wires:
  Zmin Saturation/1(Out1) -> " Currents"/4(Z10 (pu))
  1st-Order  Filter1/1 -> Product/2
  RX1/1 -> "Z1 Z0 impedances Computation "/3(Zmpu)
  psi3/1 -> Product/1
  RX5/1 -> "Z1 Z0 impedances Computation "/2(Z1maxpu)
  Tap Changer Control/1(TapNo) -> 1st-Order  Filter1/1, [Tap]
  Up/1 -> Tap Changer Control/1(Up)
  Down/1 -> Tap Changer Control/2(Down)
  Tap Changer Control/2(Ready) -> [Ready]
  Gain/1 -> " Currents"/3(Psi (deg)), [Psi]
  Trigonometric Function/1 -> Gain/1
  Product1/1 -> Trigonometric Function/1
  psi4/1 -> Product1/1
  Product/1 -> "Z1 Z0 impedances Computation "/1(k), Product1/2  "k"
  "Z1 Z0 impedances Computation "/1(Z10) -> Zmin Saturation/1(In1), Demux3/1
  B2/1 -> Gain4/1
  B1/1 -> Gain2/1  "V1"
  Demux2/1 -> Mux2/1  "VA (pu)"
  Demux2/2 -> Mux2/2  "VB (pu)"
  Demux2/3 -> Mux2/3  "VC (pu)"
  Mux2/1 -> [V1_abc]
  Gain2/1 -> Demux2/1
  Demux1/1 -> Mux1/1  "Va (pu)"
  Demux1/2 -> Mux1/2  "Vb (pu)"
  Demux1/3 -> Mux1/3  "Vc (pu)"
  Mux1/1 -> [V2_abc]
  Gain4/1 -> Demux1/1
  [V1_abc] -> " Currents"/1(V1_abc (pu))
  [V2_abc] -> " Currents"/2(V2_abc (pu))
  Demux4/1 -> Mux4/1  "IA (pu)"
  Demux4/2 -> Mux4/2  "IB (pu)"
  Demux4/3 -> Mux4/3  "IC (pu)"
  Mux4/1 -> [I1_abc]
  Demux5/1 -> Mux5/1  "Ia (pu)"
  Demux5/2 -> Mux5/2  "Ib (pu)"
  Demux5/3 -> Mux5/3  "Ic (pu)"
  Mux5/1 -> [I2_abc]
  " Currents"/1(I1_abc (pu)) -> Demux4/1
  " Currents"/2("I2_abc (pu) ") -> Demux5/1
  [I1_abc] -> Current Source/1(I1_abc)
  [I2_abc] -> Current Source/2(I2_abc)
  [V2_abc] -> Mux/2  "Vabc (cmplx) (pu)"
  Mux/1 -> m/1
  [I1_abc] -> Mux/3  "IABC (cmplx) (pu)"
  [I2_abc] -> Mux/4  "Iabc (cmplx) (pu)"
  [Tap] -> Mux/7  "Tap"
  [Z] -> Mux/5  "Z (cmplx)  (pu)"
  [V1_abc] -> Mux/1  "VABC (cmplx) (pu)"
  [Ready] -> Mux/8  "Ready"
  Demux3/1 -> Mux3/1  "Z1 (pu)"
  Demux3/2 -> Mux3/2  "Z0 (pu)"
  Mux3/1 -> [Z]
  [Psi] -> Mux/6  "Psi (degrees)"
  connections:
  Current Source/LConn3 -- B1/RConn3 -- 2*Zm/LConn3
  Current Source/LConn2 -- B1/RConn2 -- 2*Zm/LConn2
  Current Source/LConn1 -- B1/RConn1 -- 2*Zm/LConn1
  Current Source/RConn3 -- B2/LConn3 -- "2*Zm "/LConn3
  Current Source/RConn2 -- B2/LConn2 -- "2*Zm "/LConn2
  Current Source/RConn1 -- B2/LConn1 -- "2*Zm "/LConn1
  c/RConn1 -- B2/RConn3
  b/RConn1 -- B2/RConn2
  a/RConn1 -- B2/RConn1
  A/RConn1 -- B1/LConn1
  B/RConn1 -- B1/LConn2
  C/RConn1 -- B1/LConn3

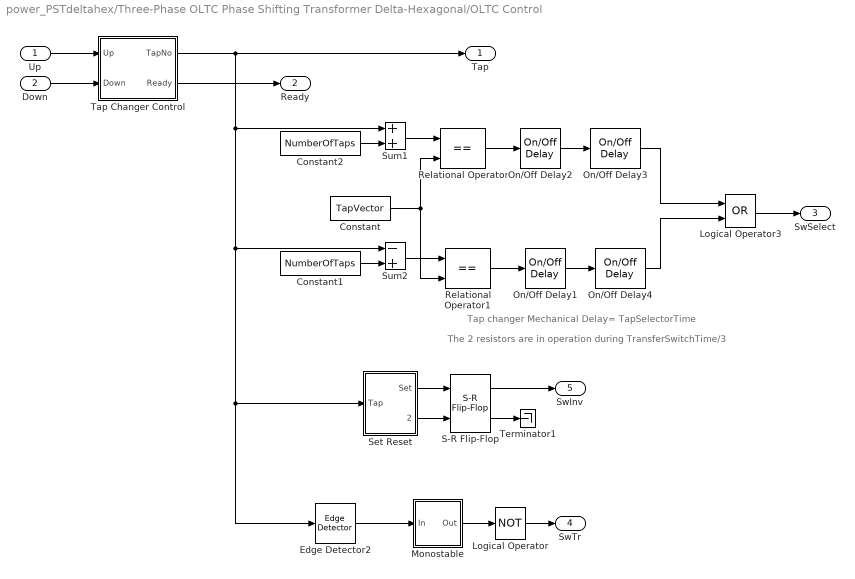
== system power_PSTdeltahex/Three-Phase OLTC Phase Shifting Transformer Delta-Hexagonal/OLTC Control ==
  note: Tap changer Mechanical Delay= TapSelectorTime
  note: The 2 resistors are in operation during TransferSwitchTime/3
  Up : Inport  Port=1  LatchInput=off
  Down : Inport  Port=2  LatchInput=off
  Constant : Constant  Value=TapVector
  Constant1 : Constant  Value=NumberOfTaps
  Constant2 : Constant  Value=NumberOfTaps
  Edge Detector2 : powerlib_extras/Control  Blocks/Edge Detector  model=Either  ic=0
  Logical Operator : Logic  Operator=NOT  AllPortsSameDT=off
  Logical Operator3 : Logic  Operator=OR  AllPortsSameDT=off
  Monostable : Subsystem  mask(Monostable Flip-Flop){EdgeDetect=Rising, t_mono=TransferSwitchTime, ic=1}
      mask prompts: EdgeDetect "Edge detection"; t_mono "Pulse duration (s):"; ic "Input at t = -eps:"
      mask help:
      | After being triggered  by the specified edge (Rising, Falling or Either), this block outputs a pulse (TRUE signal) for the time specified by parameter "Pulse duration".
      | If the specified edge is detected while the output is TRUE, the monostable is not retriggered
      |
      | The input value (0/1) at time preceeding t = 0 is specified by the parameter "input at t = -eps.
      mask init:
      | str=sprintf('%g %c',t_mono,'s');
      | if (EdgeDetect ~=3)
      |     x1 = (EdgeDetect -1)*10;
      |     x2 = (EdgeDetect -1)*30;
      | 	X1=[15-8,25,25,35+8]+0; Y1=[65+x2,65+x2,95-x2,95-x2];
      | 	X2=[15,25,35]+0;   Y2=[75+x1,85-x1,75+x1];
      | 	X3=[];X4=[];Y3=[];Y4=[];	
      | else
      | 	x1 = 10;
      | 	x2 = 30;
      | 	X1=[15,25,25,35]-14;  Y1=[65,65,95,95];
      | 	X2=[15,25,35]-14;    Y2=[75,85,75];
      | 	X3=[15,25,25,35]+14; Y3=[65+x2,65+x2,95-x2,95-x2];
      | 	X4=[15,25,35]+14;   Y4=[75+x1,85-x1,75+x1];
      | end
      mask StyleString: popup(Rising|Falling|Either),edit,edit
      mask Display:
      | plot(0,0,100,100,[100 75 75 25 25 0],[25 25 50 50 25 25]-0,X1,Y1,X2,Y2,X3,Y3,X4,Y4);
      | text(45,37,'T');
      | text(15,15,str);
  On/Off Delay1 : powerlib_extras/Control  Blocks/On//Off Delay  type_delay=On delay  delay=TransferSwitchTime/3  ic=1
  On/Off Delay2 : powerlib_extras/Control  Blocks/On//Off Delay  type_delay=On delay  delay=TransferSwitchTime/3  ic=1
  On/Off Delay3 : powerlib_extras/Control  Blocks/On//Off Delay  type_delay=Off delay  delay=2*TransferSwitchTime/3  ic=InitialStates1
  On/Off Delay4 : powerlib_extras/Control  Blocks/On//Off Delay  type_delay=Off delay  delay=2*TransferSwitchTime/3  ic=InitialStates2
  Relational Operator : RelationalOperator  Operator===
  Relational Operator1 : RelationalOperator  Operator===
  S-R Flip-Flop : simulink_extras/Flip Flops/S-R Flip-Flop  initial_condition=InitialTap>=0
  Set Reset : Subsystem
  Sum1 : Sum  SaturateOnIntegerOverflow=on
  Sum2 : Sum  Inputs=-+  SaturateOnIntegerOverflow=on
  Tap Changer Control : Subsystem  mask(Tap Changer Control){MinMaxTap=[-NumberOfTaps  +NumberOfTaps], InitialPosition=InitialTap, MecDelay=TapSelectorTime}
      mask prompts: MinMaxTap "Minimum and maximum tap number [ Min  Max ] :"; InitialPosition "Initial tap position"; MecDelay "Mechanical delay time"
      mask init:
      | if MecDelay<=0,
      | 	MecDelay=1/60;
      | end
  Terminator1 : Terminator
  Tap : Outport
  Ready : Outport  Port=2
  SwSelect : Outport  Port=3
  SwTr : Outport  Port=4
  SwInv : Outport  Port=5
  wires:
  S-R Flip-Flop/1 -> SwInv/1
  Edge Detector2/1 -> Monostable/1(In)
  Set Reset/2(Reset) -> S-R Flip-Flop/2
  Set Reset/1(Set) -> S-R Flip-Flop/1
  S-R Flip-Flop/2 -> Terminator1/1
  On/Off Delay1/1 -> On/Off Delay4/1
  Tap Changer Control/2(Ready) -> Ready/1
  Relational Operator1/1 -> On/Off Delay1/1
  Tap Changer Control/1(TapNo) -> Set Reset/1(Tap), Edge Detector2/1, Sum2/1, Sum1/1, Tap/1
  Monostable/1(Out) -> Logical Operator/1
  On/Off Delay2/1 -> On/Off Delay3/1
  Relational Operator/1 -> On/Off Delay2/1
  Up/1 -> Tap Changer Control/1(Up)
  Down/1 -> Tap Changer Control/2(Down)
  Logical Operator/1 -> SwTr/1
  Sum1/1 -> Relational Operator/1
  Constant2/1 -> Sum1/2
  Constant1/1 -> Sum2/2
  Sum2/1 -> Relational Operator1/1
  Constant/1 -> Relational Operator/2, Relational Operator1/2
  On/Off Delay3/1 -> Logical Operator3/1
  On/Off Delay4/1 -> Logical Operator3/2
  Logical Operator3/1 -> SwSelect/1

== system power_PSTdeltahex/Three-Phase OLTC Phase Shifting Transformer Delta-Hexagonal/Subsystem1 ==
  note: Delta Hexagonal Phase Shifting Transformer
  note: Each phase consists of two windings ( winding W1(no taps)  and tapped winding W2)
      | Voltage ratio= 1:1  Rated voltage of each winding=2/3*(VnomPh-Ph)
      | Two OLTCs connected to inputs (ABC) and outputs (abc)
      | select taps symmetrical with respect to center of tapped windings W2
  note: A        a
      |                  |        |
      |              A A A A A A A A A A
      |            B          W2         C
      |          B                         C
      |        B    W1                  W1   C
      |      B                                 C
      |    B                                     C
      |  +                                         +
      |    C                                     B
      | c--->C                                 B<---B
      |        C    W2                  W2   B
      |     C--->C                         B<---b
      |            C          W1         B
      |              A A A A A A A A A A

== system power_PSTdeltahex/Three-Phase OLTC Phase Shifting Transformer Delta-Hexagonal/TransfoA ==
  OLTC : Subsystem
  Transformer : Subsystem  AncestorBlock=powerlib/Elements/Multi-Winding Transformer  mask(Multi-Windings Transformer){LeftWindings=1, RightWindings=1, TappedWindings=taps on upper right winding, NumberOfTaps=19, NominalPower=[Pnom3ph/3 Fnom], NominalVoltages=Vnom_Windings, WindingResistances=Rpu_Windings, WindingInductances=Xpu_Windings, SetSaturation=off, Rm=Rmag, Lm=Lmag, Saturation=SaturationCurrentFlux, Hysteresis=off, DataFile='hysteresis.mat', Measurements=None, InitialFlux=26.7622502223547, TransfoNumber=1}
      mask prompts: LeftWindings "Number of windings on left side"; RightWindings "Number of windings on right side"; TappedWindings "Tapped winding"; NumberOfTaps "----  Number of taps (equally spaced):"; NominalPower "Nominal power and frequency [Pn(VA) fn(Hz)]:"; NominalVoltages "Winding nominal voltages [U1 U2 ... Un] (Vrms):"; WindingResistances "Winding resistances [R1 R2 ... Rn] (pu):"; WindingInductances "Winding leakage inductances [L1 L2 ... Ln] (pu):"; SetSaturation "Saturable core"; Rm "Magnetization resistance  Rm (pu)"; Lm "Magnetization reactance Lm (pu)"; Saturation "Saturation characteristic (pu) [ i1 ,  phi1 ;  i2 , phi2 ; ... ]"; Hysteresis "Simulate hysteresis"; DataFile "----  Hysteresis Data Mat file"; InitialFlux "Initial Flux (internal use)"; TransfoNumber "Device number (internal use)"
      mask init:
      | block = gcb;
      | % icon function will go here.
      | %
      | powerbase = NominalPower(1);
      | wbase = 2*pi*NominalPower(2);
      | voltbase = NominalVoltages(1);
      | BaseCurrent = (powerbase/voltbase)*sqrt(2);
      | BaseFlux = (voltbase/wbase)*sqrt(2);
      | %
      | if SetSaturation
      | 	Saturation = [-Saturation(size(Saturation,1):-1:2,:) ; Saturation(2:size(Saturation,1),:)];
      |     SaturationCurrent = [Saturation(:,1)*BaseCurrent]';
      |     SaturationFlux = [Saturation(:,2)*BaseFlux]';
      | 	if Hysteresis
      |         InitialSlope = '1';
      | 	    [Tolerances,HT,UpperFlux,LowerFlux,Current] = powericon('inithysteresis',DataFile,BaseFlux,BaseCurrent);
      | 	    if HT.UnitsPopup == 2
      | 		    % The hysteresis characteristic is in S.I.
      | 		    % consequentely we do not need to convert the in/out signals
      | 		    % of the sfunction
      | 		    BaseCurrent = 1;
      | 		    BaseFlux = 1;
      | 	    end
      | 	end
      | end
      | %
      | %powericon('NWindingsTransformerCback',block,0);
      | Ts = powericon('NWindingsTransformerInit',block);
      mask StyleString: edit,edit,popup(no taps|taps on upper left winding|taps on upper right winding),edit,edit,edit,edit,edit,checkbox,edit,edit,edit,checkbox,edit,popup(None|Winding voltages|Winding currents|Flux and excitation current ( Imag + IRm )|Flux and magnetization current ( Imag )|All measurements (V I Flux)),edit,edit
      mask CallbackString: powericon('NWindingsTransformerCback',gcb,0);|powericon('NWindingsTransformerCback',gcb,0);|powericon('NWindingsTransformerCback',gcb,1);|powericon('NWindingsTransformerCback',gcb,1);|||||powericon('NWindingsTransformerCback',gcb,0);||||powericon('NWindingsTransformerCback',gcb,0);||||
  W2- : PMIOPort  Orientation=left  Port=1  Side=Left
  W2_tap- : PMIOPort  Orientation=left  Port=2  Side=Left
  W1- : PMIOPort  Port=3  Side=Left
  W2+ : PMIOPort  Orientation=left  Port=4  Side=Right
  W2_tap+ : PMIOPort  Orientation=left  Port=5  Side=Right
  W1+ : PMIOPort  Port=6  Side=Right
  wires:
  [SwSelect] -> OLTC/1(Sw0/10)
  [SwTransfer] -> OLTC/2(SwR)
  [SwInversion] -> OLTC/3(SwInv)
  connections:
  W1-/RConn1 -- Transformer/LConn2
  W1+/RConn1 -- Transformer/LConn1
  OLTC/RConn1 -- W2_tap+/RConn1
  OLTC/RConn2 -- W2_tap-/RConn1
  Transformer/RConn1 -- OLTC/LConn1 -- W2+/RConn1
  Transformer/RConn2 -- OLTC/LConn2
  Transformer/RConn3 -- OLTC/LConn3
  Transformer/RConn4 -- OLTC/LConn4
  Transformer/RConn5 -- OLTC/LConn5
  Transformer/RConn6 -- OLTC/LConn6
  Transformer/RConn7 -- OLTC/LConn7
  Transformer/RConn8 -- OLTC/LConn8
  Transformer/RConn9 -- OLTC/LConn9
  Transformer/RConn10 -- OLTC/LConn10
  Transformer/RConn11 -- OLTC/LConn11
  Transformer/RConn12 -- OLTC/LConn12
  Transformer/RConn13 -- OLTC/LConn13
  Transformer/RConn14 -- OLTC/LConn14
  Transformer/RConn15 -- OLTC/LConn15
  Transformer/RConn16 -- OLTC/LConn16
  Transformer/RConn17 -- OLTC/LConn17
  Transformer/RConn18 -- OLTC/LConn18
  Transformer/RConn19 -- OLTC/LConn19
  Transformer/RConn20 -- OLTC/LConn20
  Transformer/RConn21 -- OLTC/LConn21 -- W2-/RConn1
